simulink model "camera"  (R2016a)
settings: Solver=FixedStepAuto  StartTime=0.0  StopTime=inf  RelTol=1e-3
libraries: SimuCopterToolbox x6, embdlinuxlib x2
settings Model: SimulationMode=external  Creator=IceDragon  LastModifiedBy=IceDragon
settings SolverCC: PositivePriorityOrder=on
settings OptimizationCC: OptimizeModelRefInitCode=on  LifeSpan=1  MaxStackSize=64
settings HardwareCC: ProdBitPerPointer=32  ProdLargestAtomicInteger=Long  ProdLargestAtomicFloat=Double  ProdWordSize=32  ProdHWDeviceType=ARM Compatible->ARM Cortex
settings RTWCC: SystemTargetFile=ert.tlc  HardwareBoard=Raspberry Pi  TemplateMakefile=ert_default_tmf  CustomInclude=bridge simucopter  CustomSource=simucopter-agent.cpp BridgeClient.cpp ZmqBridgeMessageSerializer.cpp AbstractBridgeCommandHandler.cpp BridgeMessage.cpp  CustomDefine=SIMULINK_AGENT ARDUCOPTER_NAVIO  CustomInitializer=simucopter_init();  CustomTerminator=simucopter_stop();  Toolchain=GNU GCC Raspberry Pi  BuildConfiguration=Specify  TargetLang=C++
settings CodeAppCC: ForceParamTrailComments=on  OperatorAnnotations=on  SimulinkDataObjDesc=on  SFDataObjDesc=on  MATLABFcnDesc=on  MangleLength=10  InsertBlockDesc=on  MATLABSourceComments=on
settings ERTTargetCC: SupportVariableSizeSignals=on  ExtModeMexArgs='10.66.66.254' 0 17725  RootIOFormat=Structure reference  IndentSize=4

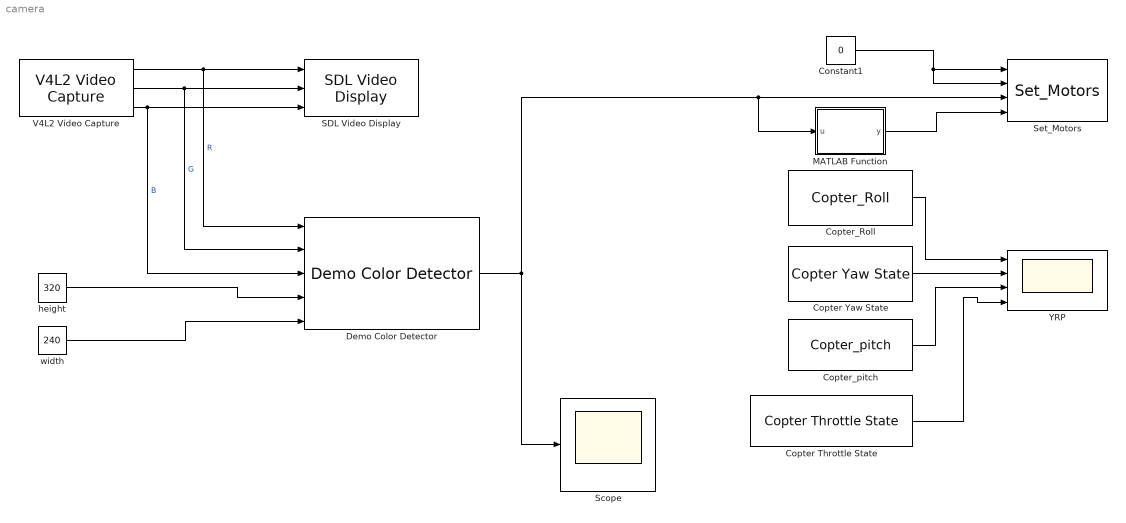
== system camera ==
  Constant1 : Constant  Value=0
  Copter Throttle State : SimuCopterToolbox/Copter Throttle State  SimulateUsing=Code generation
  Copter Yaw State : SimuCopterToolbox/Copter Yaw State  SimulateUsing=Code generation
  Copter_Roll : SimuCopterToolbox/Copter_Roll  SimulateUsing=Code generation
  Copter_pitch : SimuCopterToolbox/Copter_pitch  SimulateUsing=Code generation
  Demo Color Detector : SimuCopterToolbox/Demo Color Detector  SimulateUsing=Code generation
  MATLAB Function : MATLAB Function  TreatAsAtomicUnit=on
  SDL Video Display : embdlinuxlib/SDL Video Display  pixelFormat=RGB  pixelOrder=Planar  rowMajor=on  blockPlatform=Raspberry Pi
  Scope : Scope
  Set_Motors : SimuCopterToolbox/Set_Motors  SimulateUsing=Code generation
  V4L2 Video Capture : embdlinuxlib/V4L2 Video Capture  m_devName='/dev/video0'  roi=[0, 0, 640, 480]  imSizeSelection=320x240  imSize=[640, 480]  pixelFormat=RGB  pixelOrder=Planar  sampleTime=1/25  simOutput=Colorbars  blockPlatform=Raspberry Pi
  YRP : Scope  NumInputPorts=4
  height : Constant  Value=320
  width : Constant  Value=240
  wires:
  V4L2 Video Capture/1 -> Demo Color Detector/1, SDL Video Display/1  "R"
  V4L2 Video Capture/2 -> Demo Color Detector/2, SDL Video Display/2  "G"
  V4L2 Video Capture/3 -> Demo Color Detector/3, SDL Video Display/3  "B"
  height/1 -> Demo Color Detector/4
  width/1 -> Demo Color Detector/5
  Demo Color Detector/1 -> MATLAB Function/1(u), Set_Motors/3, Scope/1
  Copter_Roll/1 -> YRP/1
  Copter_pitch/1 -> YRP/3
  Copter Yaw State/1 -> YRP/2
  Copter Throttle State/1 -> YRP/4
  Constant1/1 -> Set_Motors/1, Set_Motors/2
  MATLAB Function/1(y) -> Set_Motors/4

== matlab function camera/MATLAB Function ==
  data: u input; y output
function y = fcn(u)
%#codegen
if (u == 0)
    y = 0;
else
    y = 0.1;
end
end
